simulink model "complex_example"  (R2024b)
settings: Solver=VariableStepAuto  StartTime=0.0  StopTime=10.0  RelTol=1e-3
settings Model: Creator=Stefania  LastModifiedBy=Stefania

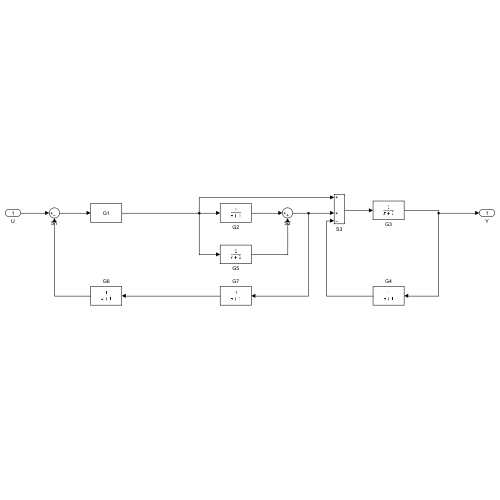
[thumbnail: Simulink's stored preview of the top-level diagram]
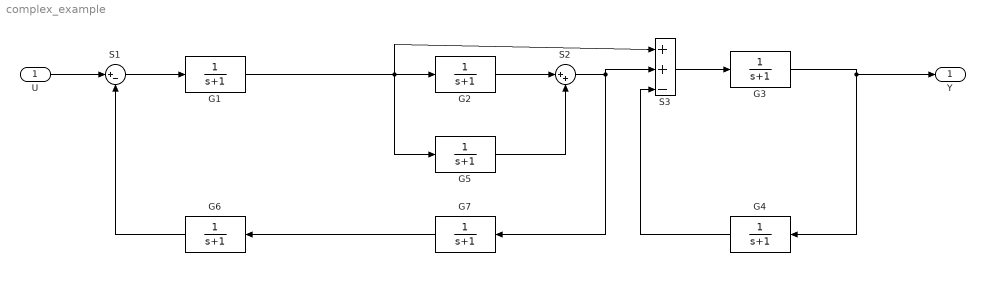
== system complex_example ==
  U : Inport
  G{1..7} (7 alike) : TransferFcn  Denominator=[1 1]
      G1 mask Display: disp('G1')
  S1 : Sum  Inputs=|+-
  S2 : Sum  Inputs=|++
  S3 : Sum  Inputs=+|+-
  Y : Outport
  wires:
  U/1 -> S1/1
  S1/1 -> G1/1
  G1/1 -> G5/1, G2/1, S3/1
  S3/1 -> G3/1
  G3/1 -> Y/1, G4/1
  G6/1 -> S1/2
  G2/1 -> S2/1
  G5/1 -> S2/2
  S2/1 -> G7/1, S3/2
  G4/1 -> S3/3
  G7/1 -> G6/1
